simulink model "Projet_EBD_ABS"  (R2022b)
settings: Solver=VariableStepAuto  StartTime=0.0  StopTime=15  RelTol=1e-3
undefined symbols (not defined in the file): gp, J, m, rR, V0, w0
libraries: simulink x2, slpidlib x1
settings Model: Creator=elmeh  LastModifiedBy=elmeh
settings SolverCC: ZeroCrossAlgorithm=Adaptive
settings DebuggingCC: IgnoredZcDiagnostic=none

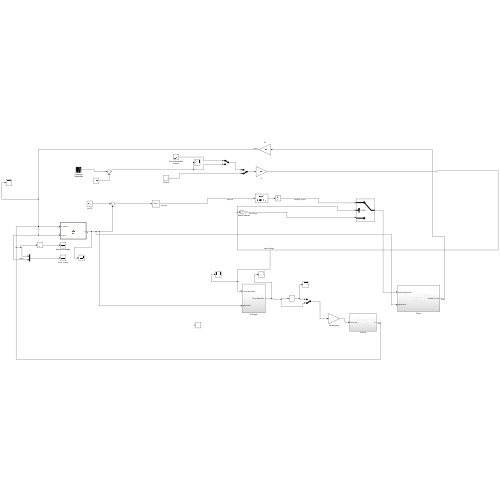
[thumbnail: Simulink's stored preview of the top-level diagram]
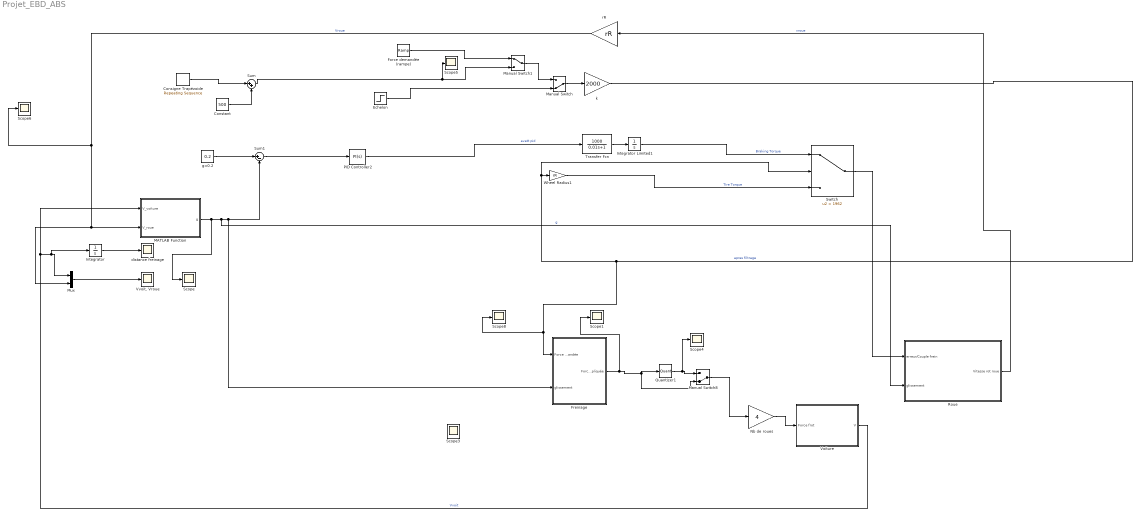
== system Projet_EBD_ABS ==
  Consigne Trapézoide : simulink/Sources/Repeating Sequence  rep_seq_t=[0 0.1 0.2 0.3 0.4 0.5]  rep_seq_y=[0 1000 1000 1000 0 0]
  Constant : Constant  Value=500
  Echelon : Step  SampleTime=0
  Force demandée (rampe) : simulink/Sources/Ramp  slope=1  start=0  InitialOutput=0
  Freinage : Subsystem
  Integrator : Integrator  LimitOutput=on  LowerSaturationLimit=0
  Integrator Limited1 : Integrator  LimitOutput=on  UpperSaturationLimit=1500  LowerSaturationLimit=0
  MATLAB Function : MATLAB Function  TreatAsAtomicUnit=on
  Manual Switch : ManualSwitch  CurrentSetting=0
  Manual Switch1 : ManualSwitch
  Manual Switch8 : ManualSwitch  CurrentSetting=0
  Mux : Mux  Inputs=2
  Nb de roues : Gain  Gain=4
  PID Controller2 : slpidlib/PID Controller  Controller=PI  Form=Parallel  TimeDomain=Continuous-time  UseExternalTs=off  SampleTime=-1  IntegratorMethod=Forward Euler  FilterMethod=Forward Euler  ControllerParametersSource=internal  P=50  I=1  UseKiTs=off  D=0.0001  N=1  UseFilter=on  TunerSelectOption=Transfer Function Based (PID Tuner App)  InitialConditionSource=internal  InitialConditionForIntegrator=0  InitialConditionForFilter=0  DifferentiatorICPrevScaledInput=0  ExternalReset=none  TrackingMode=off  Kt=1  LimitOutput=off  SatLimitsSource=internal  UpperSaturationLimit=inf  LowerSaturationLimit=-inf  LinearizeAsGain=on  AntiWindupMode=none  Kb=1  LimitIntegrator=off  UpperIntegratorSaturationLimit=inf  LowerIntegratorSaturationLimit=-inf  POutMin=[]  POutMax=[]  IOutMin=[]  IOutMax=[]  DOutMin=[]  DOutMax=[]  NOutMin=[]  NOutMax=[]  SumOutMin=[]  SumOutMax=[]  SaturationOutMin=[]  SaturationOutMax=[]  PParamMin=[]  PParamMax=[]  IParamMin=[]  IParamMax=[]  DParamMin=[]  DParamMax=[]  NParamMin=[]  NParamMax=[]  KbParamMin=[]  KbParamMax=[]  KtParamMin=[]  KtParamMax=[]  KbOutMin=[]  KbOutMax=[]  KtOutMin=[]  KtOutMax=[]  IntegratorOutMin=[]  IntegratorOutMax=[]  FilterOutMin=[]  FilterOutMax=[]  SumI1OutMin=[]  SumI1OutMax=[]  SumI2OutMin=[]  SumI2OutMax=[]  SumI3OutMin=[]  SumI3OutMax=[]  SumI4OutMin=[]  SumI4OutMax=[]  SumDOutMin=[]  SumDOutMax=[]  DifferentiatorOutMin=[]  DifferentiatorOutMax=[]  FilterDiffOutCoefMin=[]  FilterDiffOutCoefMax=[]  ReciprocalOutMin=[]  ReciprocalOutMax=[]  SumDenOutMin=[]  SumDenOutMax=[]  SumNumOutMin=[]  SumNumOutMax=[]  DivideOutMin=[]  DivideOutMax=[]  UdiffTsProdOutMin=[]  UdiffTsProdOutMax=[]  NTsProdOutMin=[]  NTsProdOutMax=[]  UintegralTsProdOutMin=[]  UintegralTsProdOutMax=[]  UngainTsProdOutMin=[]  UngainTsProdOutMax=[]  ClampingZeroOutDataTypeStr=Inherit: Inherit via back propagation  ClampingZeroOutMin=[]  ClampingZeroOutMax=[]  FilterDenConstantOutDataTypeStr=Inherit: Inherit via back propagation  FilterDenConstantOutMin=[]  FilterDenConstantOutMax=[]  PCopyOutDataTypeStr=Inherit: Inherit via back propagation  PCopyOutMin=[]  PCopyOutMax=[]  NCopyOutDataTypeStr=Inherit: Inherit via back propagation  NCopyOutMin=[]  NCopyOutMax=[]  IntegratorContinuousStateAttributes=''  IntegratorStateMustResolveToSignalObject=off  IntegratorRTWStateStorageClass=Auto  FilterContinuousStateAttributes=''  FilterStateMustResolveToSignalObject=off  FilterRTWStateStorageClass=Auto  ParallelPVariant=InternalParameters  IdealPVariant=Disabled  IVariant=InternalParameters  DVariant=Disabled  IntegratorVariant=Continuous  SatVariant=Disabled  AWVariant=Passthrough  PCopyVariant=Disabled  TRVariant=Disabled  FdbkBlocksVariant=Forward  IdealPFdbkVariant=Disabled  SatFdbkVariant=Disabled  DerivativeFilterVariant=Disabled  NVariant=Disabled  NCopyVariant=Disabled_SignalSpec  FilterICVariant=Disabled  IntegratorICVariant=InternalICs  ExternalResetVariant=Disabled  TRSumVariant=Passthrough  SumFdbkVariant=Disabled  SumVariant=Sum_PI  TsampFilterVariant=InternalTs  TsampNgainVariant=Passthrough  TsampIntegralVariant=Passthrough  ExternalSaturationOutDataTypeStr=Inherit: Same as second input
  Quantizer1 : Quantizer  QuantizationInterval=400
  Roue : Subsystem
  Scope{,1,3..6,8} (7 alike) : Scope
  Sum : Sum  Inputs=|++
  Sum1 : Sum  Inputs=|+-
  Switch : Switch  Criteria=u2 > Threshold  Threshold=1962  SaturateOnIntegerOverflow=off  InputSameDT=off
  Transfer Fcn : TransferFcn  Numerator=[1000]  Denominator=[0.01 1]
  Voiture : Subsystem
  "Vvoit, Vroue" : Scope
  Wheel Radius1 : Gain  Gain=rR
  distance freinage : Scope
  g=0.2 : Constant  Value=0.2
  k : Gain  Gain=2000
  rR : Gain  Gain=rR
  wires:
  Force demandée (rampe)/1 -> Manual Switch1/1
  Echelon/1 -> Manual Switch/2
  Manual Switch1/1 -> Manual Switch/1
  Sum/1 -> Scope5/1, Manual Switch1/2
  Nb de roues/1 -> Voiture/1(Force frot)
  Manual Switch/1 -> k/1
  Roue/1(Vitesse rot roue) -> rR/1  "vroue"
  rR/1 -> Scope6/1, Mux/2, MATLAB Function/2(V_roue)  "Vroue"
  Mux/1 -> "Vvoit, Vroue"/1
  Voiture/1("V ") -> Integrator/1, Mux/1, MATLAB Function/1(V_voiture)  "Vvoit"
  Integrator/1 -> distance freinage/1
  k/1 -> Switch/2, Wheel Radius1/1, Scope8/1, Freinage/1(Force demandée)  "apres filtrage"
  Freinage/1("Force Appliquée ") -> Manual Switch8/2, Quantizer1/1, Scope1/1
  Quantizer1/1 -> Scope4/1, Manual Switch8/1
  Manual Switch8/1 -> Nb de roues/1
  Consigne Trapézoide/1 -> Sum/1
  Constant/1 -> Sum/2
  g=0.2/1 -> Sum1/1
  MATLAB Function/1(g) -> Roue/2(glissement), Freinage/2("glissement "), Sum1/2, Scope/1  "g"
  Sum1/1 -> PID Controller2/1
  Wheel Radius1/1 -> Switch/3  "Tire Torque"
  Switch/1 -> Roue/1(erreur/Couple frein)
  Transfer Fcn/1 -> Integrator Limited1/1
  Integrator Limited1/1 -> Switch/1  "Braking Torque"
  PID Controller2/1 -> Transfer Fcn/1  "avatt pid"

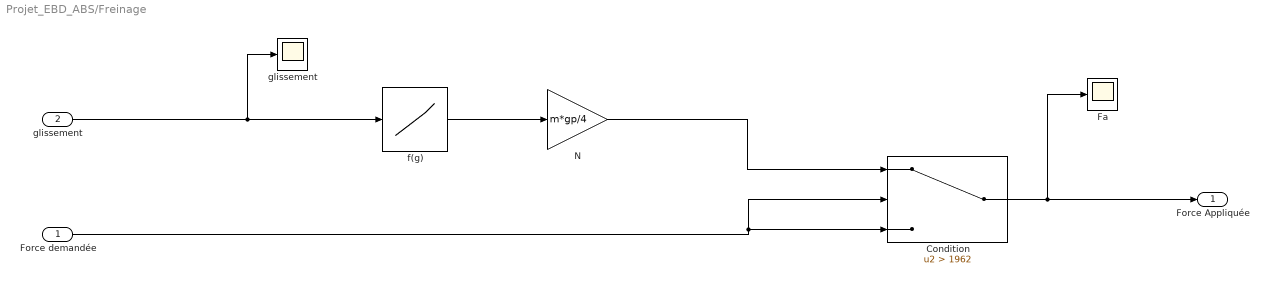
== system Projet_EBD_ABS/Freinage ==
  Force demandée : Inport
  "glissement " : Inport  Port=2
  "Condition " : Switch  Criteria=u2 > Threshold  Threshold=1962  SaturateOnIntegerOverflow=off  InputSameDT=off
  "Fa " : Scope
  N : Gain  Gain=m*gp/4
  f(g) : Lookup_n-D  NumberOfTableDimensions=1  BreakpointsForDimension1=[0,0.1,0.2,0.3,0.4,0.5,0.6,0.7,0.8,0.9,1.0]  Table=[0.0,0.85,0.95,0.78,0.73,0.7,0.68,0.66,0.64,0.62,0.61]  InternalRulePriority=Speed  RndMeth=Simplest
  glissement : Scope
  "Force Appliquée " : Outport  VectorParamsAs1DForOutWhenUnconnected=off
  wires:
  f(g)/1 -> N/1
  Force demandée/1 -> "Condition "/3, "Condition "/2
  "glissement "/1 -> f(g)/1, glissement/1
  "Condition "/1 -> "Force Appliquée "/1, "Fa "/1
  N/1 -> "Condition "/1

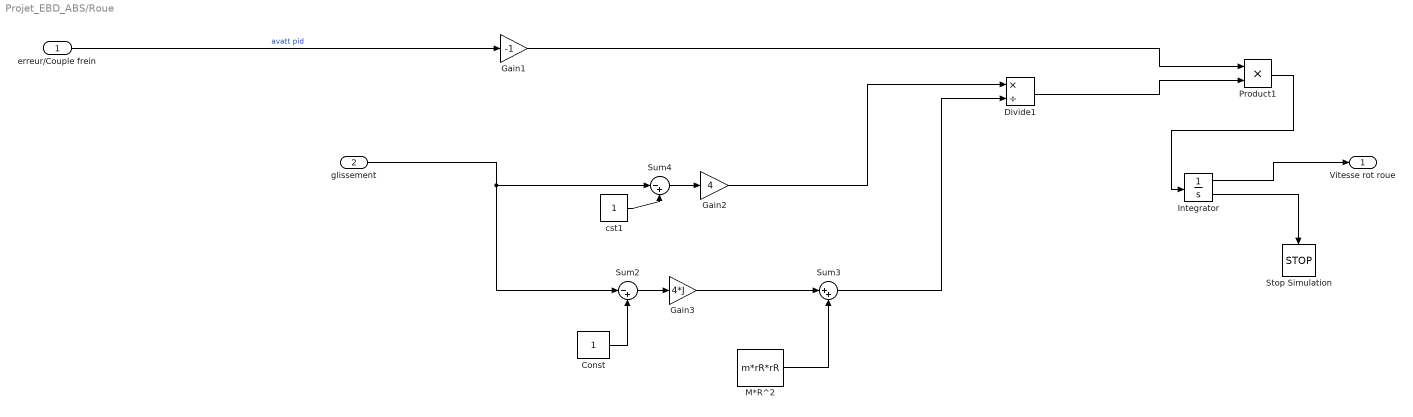
== system Projet_EBD_ABS/Roue ==
  erreur/Couple frein : Inport
  glissement : Inport  Port=2
  Const : Constant
  Divide1 : Product  Inputs=*/
  Gain1 : Gain  Gain=-1
  Gain2 : Gain  Gain=4
  Gain3 : Gain  Gain=4*J
  Integrator : Integrator  InitialCondition=w0  LimitOutput=on  LowerSaturationLimit=0  ShowSaturationPort=on
  M*R^2 : Constant  Value=m*rR*rR
  Product1 : Product
  Stop Simulation : Stop
  Sum2 : Sum  Inputs=|-+
  Sum3 : Sum  Inputs=|++
  Sum4 : Sum  Inputs=|-+
  cst1 : Constant
  Vitesse rot roue : Outport
  wires:
  Integrator/2 -> Stop Simulation/1
  Product1/1 -> Integrator/1
  glissement/1 -> Sum2/1, Sum4/1
  Const/1 -> Sum2/2
  M*R^2/1 -> Sum3/2
  Sum3/1 -> Divide1/2
  Gain2/1 -> Divide1/1
  Gain1/1 -> Product1/1
  Sum2/1 -> Gain3/1
  Sum4/1 -> Gain2/1
  Divide1/1 -> Product1/2
  Gain3/1 -> Sum3/1
  cst1/1 -> Sum4/2
  Integrator/1 -> Vitesse rot roue/1
  erreur/Couple frein/1 -> Gain1/1  "avatt pid"

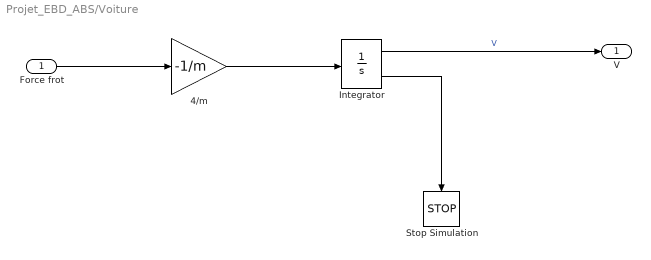
== system Projet_EBD_ABS/Voiture ==
  Force frot : Inport
  4/m : Gain  Gain=-1/m
  Integrator : Integrator  InitialCondition=V0  LimitOutput=on  LowerSaturationLimit=0  ShowSaturationPort=on
  Stop Simulation : Stop
  "V " : Outport
  wires:
  Force frot/1 -> 4/m/1
  4/m/1 -> Integrator/1
  Integrator/1 -> "V "/1  "V"
  Integrator/2 -> Stop Simulation/1

== matlab function Projet_EBD_ABS/MATLAB Function ==
  data: V_voiture input; V_roue input; g output
function g = fcn(V_voiture,V_roue)

g = (V_voiture - V_roue)/V_voiture;
